simulink model "ddc_bpm_476_066"  (Simulink 7.8)
settings: Solver=ode45  StartTime=0.0  StopTime=0.012  RelTol=1e-3
undefined symbols (not defined in the file): dt_sim, frev_476, Fs_adc, xlipgetpartsetting
libraries: xbsIndex_r4 x601, simulink x5
(part 4 of 6)

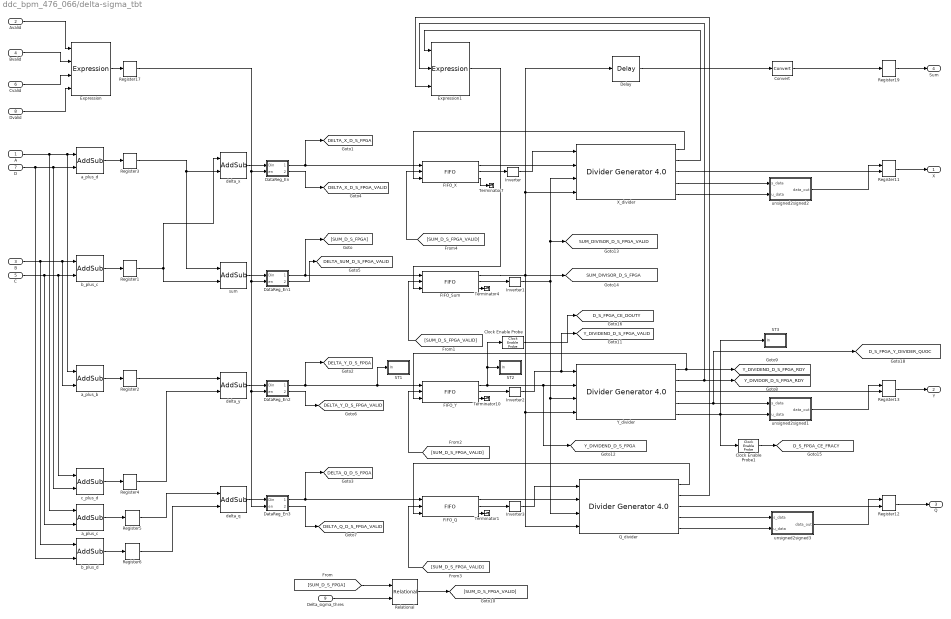
== system ddc_bpm_476_066/delta-sigma_tbt ==
  A : Inport
  Avalid : Inport  Port=2
  B : Inport  Port=3
  Bvalid : Inport  Port=4
  C : Inport  Port=5
  Cvalid : Inport  Port=6
  D : Inport  Port=7
  Dvalid : Inport  Port=8
  Delta_sigma_thres : Inport  Port=9
  Clock Enable Probe : xbsIndex_r4/Clock Enable Probe  inherit_constraints=on  block_type=ceprobe
      settings: infoedit="Clock enable extractor.  Produces a Boolean output that mirrors the hardware clock enable associated with the input sample rate.<br><br>Hardware notes: in hardware this block costs nothing."
  Clock Enable Probe1 : xbsIndex_r4/Clock Enable Probe  inherit_constraints=on  block_type=ceprobe
      settings: infoedit="Clock enable extractor.  Produces a Boolean output that mirrors the hardware clock enable associated with the input sample rate.<br><br>Hardware notes: in hardware this block costs nothing."
  Convert : xbsIndex_r4/Convert  gui_display_data_type=Fixed-point  arith_type="Signed  (2's comp)"  n_bits=24  bin_pt=20  float_type=Single  exp_bits=8  fraction_bits=24  quantization="Round  (unbiased: +/- Inf)"  overflow=Flag as error  en=off  latency=0  dbl_ovrd=off  pipeline=off  block_type=convert
  DataReg_En : Subsystem
  DataReg_En1 : Subsystem
  DataReg_En2 : Subsystem
  DataReg_En3 : Subsystem
  Delay : xbsIndex_r4/Delay  rst=off  infoeditControl=Selection of Reset will increase slice count due to use of real FFs and instead of SRLs  en=off  latency=39  dbl_ovrd=off  reg_retiming=off  block_type=delay
  Expression : xbsIndex_r4/Expression  expression=a & b & c & d  align_bp=on  en=off  latency=0  precision=Full  arith_type=Unsigned  n_bits=16  bin_pt=0  dbl_ovrd=off  block_type=expr
  Expression1 : xbsIndex_r4/Expression  expression=a & b & c  align_bp=on  en=off  latency=0  precision=Full  arith_type=Unsigned  n_bits=16  bin_pt=0  dbl_ovrd=off  block_type=expr
  FIFO_Q : xbsIndex_r4/FIFO  performance_options=First_Word_Fall_Through  depth=32  percent_nbits=1  rst=off  en=off  use_dcount=off  use_percent_full_port=off  use_almost_empty=off  almost_empty_thresh=2  use_almost_full=off  almost_full_thresh=14  dbl_ovrd=off  mem_type=Distributed RAM  explicit_period=off  block_type=fifo
  FIFO_Sum : xbsIndex_r4/FIFO  performance_options=First_Word_Fall_Through  depth=32  percent_nbits=1  rst=off  en=off  use_dcount=off  use_percent_full_port=off  use_almost_empty=off  almost_empty_thresh=2  use_almost_full=off  almost_full_thresh=14  dbl_ovrd=off  mem_type=Distributed RAM  explicit_period=off  block_type=fifo
  FIFO_X : xbsIndex_r4/FIFO  performance_options=First_Word_Fall_Through  depth=32  percent_nbits=1  rst=off  en=off  use_dcount=off  use_percent_full_port=off  use_almost_empty=off  almost_empty_thresh=2  use_almost_full=off  almost_full_thresh=14  dbl_ovrd=off  mem_type=Distributed RAM  explicit_period=off  block_type=fifo
  FIFO_Y : xbsIndex_r4/FIFO  performance_options=First_Word_Fall_Through  depth=32  percent_nbits=1  rst=off  en=off  use_dcount=off  use_percent_full_port=off  use_almost_empty=off  almost_empty_thresh=2  use_almost_full=off  almost_full_thresh=14  dbl_ovrd=off  mem_type=Distributed RAM  explicit_period=off  block_type=fifo
  Inverter{,1..3} (4 alike) : xbsIndex_r4/Inverter  en=off  latency=0  dbl_ovrd=off  block_type=inv
  Q_divider : xbsIndex_r4/Divider Generator 4.0   algorithm_type=High_Radix  remainder_type=Fractional  fractional_width=23  clocks_per_division=1  divide_by_zero_detect=off  flowcontrol=NonBlocking  optimizegoal=Performance  latency_configuration=Automatic  latency=39  dividend_has_tuser=off  dividend_has_tlast=off  divisor_has_tuser=off  divisor_has_tlast=off  aclken=off  aresetn=off  outtready=off  outtlastbehv=Null  trim_axipin_name=on  dividend_tuser_width=1  divisor_tuser_width=1  operand_sign=Signed  dividend_and_quotient_width=16  divisor_width=16  ip_name=Divider Generator  ip_version=4.0  dsptool_ready=true  ipcore_usecache=true  ipcore_useipmodelcache=true  wrapper_available=true  port_translation_map={'aclken' => 'en','aresetn' => 'rst'}  ipcore_fpga_part=xlipgetpartsetting(gcb, {'virtex7', 'xc7v1500t', '-2', 'fhg1157'})  ipcore_verbose=false  block_type=div_gen_v4_0
      settings: infoedit=Divider Generator 4.0
  Register{1..6,17,19} (8 alike) : xbsIndex_r4/Register  init=0  rst=off  en=off  dbl_ovrd=off  block_type=register
  Register11 : xbsIndex_r4/Register  init=0  rst=off  en=on  dbl_ovrd=off  block_type=register
  Register12 : xbsIndex_r4/Register  init=0  rst=off  en=on  dbl_ovrd=off  block_type=register
  Register13 : xbsIndex_r4/Register  init=0  rst=off  en=on  dbl_ovrd=off  block_type=register
  Relational : xbsIndex_r4/Relational  mode=a>b  en=off  latency=0  dbl_ovrd=off  block_type=relational
  ST1 : Subsystem
  ST2 : Subsystem
  ST3 : Subsystem
  Terminator{1,4,7,10} (4 alike) : Terminator
  X_divider : xbsIndex_r4/Divider Generator 4.0   algorithm_type=High_Radix  remainder_type=Fractional  fractional_width=23  clocks_per_division=1  divide_by_zero_detect=off  flowcontrol=NonBlocking  optimizegoal=Performance  latency_configuration=Automatic  latency=39  dividend_has_tuser=off  dividend_has_tlast=off  divisor_has_tuser=off  divisor_has_tlast=off  aclken=off  aresetn=off  outtready=off  outtlastbehv=Null  trim_axipin_name=on  dividend_tuser_width=1  divisor_tuser_width=1  operand_sign=Signed  dividend_and_quotient_width=16  divisor_width=16  ip_name=Divider Generator  ip_version=4.0  dsptool_ready=true  ipcore_usecache=true  ipcore_useipmodelcache=true  wrapper_available=true  port_translation_map={'aclken' => 'en','aresetn' => 'rst'}  ipcore_fpga_part=xlipgetpartsetting(gcb, {'virtex7', 'xc7v1500t', '-2', 'fhg1157'})  ipcore_verbose=false  block_type=div_gen_v4_0
      settings: infoedit=Divider Generator 4.0
  Y_divider : xbsIndex_r4/Divider Generator 4.0   algorithm_type=High_Radix  remainder_type=Fractional  fractional_width=23  clocks_per_division=1  divide_by_zero_detect=off  flowcontrol=NonBlocking  optimizegoal=Performance  latency_configuration=Automatic  latency=39  dividend_has_tuser=off  dividend_has_tlast=off  divisor_has_tuser=off  divisor_has_tlast=off  aclken=off  aresetn=off  outtready=off  outtlastbehv=Null  trim_axipin_name=on  dividend_tuser_width=1  divisor_tuser_width=1  operand_sign=Signed  dividend_and_quotient_width=16  divisor_width=16  ip_name=Divider Generator  ip_version=4.0  dsptool_ready=true  ipcore_usecache=true  ipcore_useipmodelcache=true  wrapper_available=true  port_translation_map={'aclken' => 'en','aresetn' => 'rst'}  ipcore_fpga_part=xlipgetpartsetting(gcb, {'virtex7', 'xc7v1500t', '-2', 'fhg1157'})  ipcore_verbose=false  block_type=div_gen_v4_0
      settings: infoedit=Divider Generator 4.0
  a_plus_b : xbsIndex_r4/AddSub  mode=Addition  use_carryin=off  use_carryout=off  en=off  latency=0  precision=Full  arith_type=Unsigned  n_bits=16  bin_pt=14  quantization=Truncate  overflow=Wrap  dbl_ovrd=off  use_behavioral_HDL=off  hw_selection=Fabric  pipelined=off  block_type=addsub
  a_plus_c : xbsIndex_r4/AddSub  mode=Addition  use_carryin=off  use_carryout=off  en=off  latency=0  precision=Full  arith_type=Unsigned  n_bits=16  bin_pt=14  quantization=Truncate  overflow=Wrap  dbl_ovrd=off  use_behavioral_HDL=off  hw_selection=Fabric  pipelined=off  block_type=addsub
  a_plus_d : xbsIndex_r4/AddSub  mode=Addition  use_carryin=off  use_carryout=off  en=off  latency=0  precision=Full  arith_type=Unsigned  n_bits=16  bin_pt=14  quantization=Truncate  overflow=Wrap  dbl_ovrd=off  use_behavioral_HDL=off  hw_selection=Fabric  pipelined=off  block_type=addsub
  b_plus_c : xbsIndex_r4/AddSub  mode=Addition  use_carryin=off  use_carryout=off  en=off  latency=0  precision=Full  arith_type=Unsigned  n_bits=16  bin_pt=14  quantization=Truncate  overflow=Wrap  dbl_ovrd=off  use_behavioral_HDL=off  hw_selection=Fabric  pipelined=off  block_type=addsub
  b_plus_d : xbsIndex_r4/AddSub  mode=Addition  use_carryin=off  use_carryout=off  en=off  latency=0  precision=Full  arith_type=Unsigned  n_bits=16  bin_pt=14  quantization=Truncate  overflow=Wrap  dbl_ovrd=off  use_behavioral_HDL=off  hw_selection=Fabric  pipelined=off  block_type=addsub
  c_plus_d : xbsIndex_r4/AddSub  mode=Addition  use_carryin=off  use_carryout=off  en=off  latency=0  precision=Full  arith_type=Unsigned  n_bits=16  bin_pt=14  quantization=Truncate  overflow=Wrap  dbl_ovrd=off  use_behavioral_HDL=off  hw_selection=Fabric  pipelined=off  block_type=addsub
  delta_q : xbsIndex_r4/AddSub  mode=Subtraction  use_carryin=off  use_carryout=off  en=off  latency=0  precision=Full  arith_type=Unsigned  n_bits=16  bin_pt=14  quantization=Truncate  overflow=Wrap  dbl_ovrd=off  use_behavioral_HDL=off  hw_selection=Fabric  pipelined=off  block_type=addsub
  delta_x : xbsIndex_r4/AddSub  mode=Subtraction  use_carryin=off  use_carryout=off  en=off  latency=0  precision=Full  arith_type=Unsigned  n_bits=16  bin_pt=14  quantization=Truncate  overflow=Wrap  dbl_ovrd=off  use_behavioral_HDL=off  hw_selection=Fabric  pipelined=off  block_type=addsub
  delta_y : xbsIndex_r4/AddSub  mode=Subtraction  use_carryin=off  use_carryout=off  en=off  latency=0  precision=Full  arith_type=Unsigned  n_bits=16  bin_pt=14  quantization=Truncate  overflow=Wrap  dbl_ovrd=off  use_behavioral_HDL=off  hw_selection=Fabric  pipelined=off  block_type=addsub
  sum : xbsIndex_r4/AddSub  mode=Addition  use_carryin=off  use_carryout=off  en=off  latency=0  precision=Full  arith_type=Unsigned  n_bits=16  bin_pt=14  quantization=Truncate  overflow=Wrap  dbl_ovrd=off  use_behavioral_HDL=off  hw_selection=Fabric  pipelined=off  block_type=addsub
  unsigned2signed1 : Subsystem
  unsigned2signed2 : Subsystem
  unsigned2signed3 : Subsystem
  X : Outport
  Y : Outport  Port=2
  Q : Outport  Port=3
  Sum : Outport  Port=4
  tag scope: DELTA_Q_D_S_FPGA=global, DELTA_Q_D_S_FPGA_VALID=global, DELTA_SUM_D_S_FPGA_VALID=global, DELTA_X_D_S_FPGA=global, DELTA_X_D_S_FPGA_VALID=global, DELTA_Y_D_S_FPGA=global, DELTA_Y_D_S_FPGA_VALID=global, D_S_FPGA_CE_DOUTY=global, D_S_FPGA_CE_FRACY=global, D_S_FPGA_Y_DIVIDER_QUOC=global, SUM_DIVISOR_D_S_FPGA=global, SUM_DIVISOR_D_S_FPGA_VALID=global, Y_DIVIDEND_D_S_FPGA=global, Y_DIVIDEND_D_S_FPGA_RDY=global, Y_DIVIDEND_D_S_FPGA_VALID=global, Y_DIVIDOR_D_S_FPGA_RDY=global
  wires:
  A/1 -> a_plus_d/1, a_plus_b/1, a_plus_c/1
  D/1 -> a_plus_d/2, c_plus_d/2, b_plus_d/2
  B/1 -> b_plus_c/1, a_plus_b/2, b_plus_d/1
  C/1 -> b_plus_c/2, c_plus_d/1, a_plus_c/2
  a_plus_d/1 -> Register3/1
  b_plus_c/1 -> Register1/1
  a_plus_b/1 -> Register2/1
  c_plus_d/1 -> Register4/1
  a_plus_c/1 -> Register5/1
  b_plus_d/1 -> Register6/1
  Register3/1 -> sum/1, delta_x/2
  Register1/1 -> sum/2, delta_x/1
  Register2/1 -> delta_y/1
  Register4/1 -> delta_y/2
  Register5/1 -> delta_q/1
  Register6/1 -> delta_q/2
  delta_q/1 -> DataReg_En3/1(Din)
  delta_x/1 -> DataReg_En/1(Din)
  Register19/1 -> Sum/1
  Avalid/1 -> Expression/1
  Bvalid/1 -> Expression/2
  Cvalid/1 -> Expression/3
  Dvalid/1 -> Expression/4
  Expression/1 -> Register17/1
  DataReg_En1/1(Dout) -> [SUM_D_S_FPGA], FIFO_Sum/1
  Register17/1 -> DataReg_En/2(en), DataReg_En1/2(en), DataReg_En2/2(en), DataReg_En3/2(en)
  Register13/1 -> Y/1
  Register11/1 -> X/1
  Register12/1 -> Q/1
  sum/1 -> DataReg_En1/1(Din)
  delta_y/1 -> DataReg_En2/1(Din)
  DataReg_En1/2(Valid) -> [DELTA_SUM_D_S_FPGA_VALID]
  Delay/1 -> Convert/1
  X_divider/3 -> Register11/2
  DataReg_En/1(Dout) -> [DELTA_X_D_S_FPGA], FIFO_X/1
  DataReg_En/2(Valid) -> [DELTA_X_D_S_FPGA_VALID]
  Y_divider/5 -> ST3/1(In), Clock Enable Probe1/1, unsigned2signed1/2(u_data)
  Y_divider/3 -> Register13/2
  Q_divider/3 -> Register12/2
  DataReg_En2/1(Dout) -> [DELTA_Y_D_S_FPGA], FIFO_Y/1, ST1/1(In)
  DataReg_En2/2(Valid) -> [DELTA_Y_D_S_FPGA_VALID]
  DataReg_En3/1(Dout) -> [DELTA_Q_D_S_FPGA], FIFO_Q/1
  DataReg_En3/2(Valid) -> [DELTA_Q_D_S_FPGA_VALID]
  X_divider/2 -> Expression1/1
  Y_divider/1 -> [Y_DIVIDEND_D_S_FPGA_RDY], FIFO_Y/3
  Y_divider/2 -> [Y_DIVIDOR_D_S_FPGA_RDY], Expression1/2
  Delta_sigma_thres/1 -> Relational/2
  [SUM_D_S_FPGA] -> Relational/1
  Relational/1 -> [SUM_D_S_FPGA_VALID]
  [SUM_D_S_FPGA_VALID] -> FIFO_Sum/2
  FIFO_Sum/1 -> Y_divider/4, Q_divider/4, X_divider/4, Delay/1, [SUM_DIVISOR_D_S_FPGA]
  FIFO_X/1 -> X_divider/2
  FIFO_Q/1 -> Q_divider/2
  FIFO_Y/1 -> Y_divider/2, [Y_DIVIDEND_D_S_FPGA], ST2/1(In), Clock Enable Probe/1
  Q_divider/2 -> Expression1/3
  Expression1/1 -> FIFO_Sum/3
  X_divider/1 -> FIFO_X/3
  Q_divider/1 -> FIFO_Q/3
  [SUM_D_S_FPGA_VALID] -> FIFO_Y/2
  [SUM_D_S_FPGA_VALID] -> FIFO_Q/2
  FIFO_Q/2 -> Inverter3/1
  FIFO_Q/3 -> Terminator1/1
  FIFO_Sum/2 -> Inverter1/1
  FIFO_Sum/3 -> Terminator4/1
  FIFO_X/3 -> Terminator7/1
  FIFO_Y/2 -> Inverter2/1
  FIFO_Y/3 -> Terminator10/1
  [SUM_D_S_FPGA_VALID] -> FIFO_X/2
  FIFO_X/2 -> Inverter/1
  Inverter/1 -> X_divider/1
  Inverter1/1 -> Y_divider/3, Q_divider/3, X_divider/3, [SUM_DIVISOR_D_S_FPGA_VALID]
  Inverter2/1 -> Y_divider/1, [Y_DIVIDEND_D_S_FPGA_VALID]
  Inverter3/1 -> Q_divider/1
  Clock Enable Probe1/1 -> [D_S_FPGA_CE_FRACY]
  Clock Enable Probe/1 -> [D_S_FPGA_CE_DOUTY]
  X_divider/5 -> unsigned2signed2/2(u_data)
  X_divider/4 -> unsigned2signed2/1(s_data)
  unsigned2signed2/1(data_out) -> Register11/1
  Y_divider/4 -> [D_S_FPGA_Y_DIVIDER_QUOC], unsigned2signed1/1(s_data)
  unsigned2signed1/1(data_out) -> Register13/1
  Q_divider/5 -> unsigned2signed3/2(u_data)
  Q_divider/4 -> unsigned2signed3/1(s_data)
  unsigned2signed3/1(data_out) -> Register12/1
  Convert/1 -> Register19/1

== system ddc_bpm_476_066/BPF/Cast ==
  data_in : Inport
  en : Inport  Port=2
  Convert : xbsIndex_r4/Convert  gui_display_data_type=Fixed-point  arith_type="Signed  (2's comp)"  n_bits=24  bin_pt=22  float_type=Single  exp_bits=8  fraction_bits=24  quantization="Round  (unbiased: +/- Inf)"  overflow=Flag as error  en=off  latency=0  dbl_ovrd=off  pipeline=off  block_type=convert
      settings: xl_area=[0, 0, 0, 0, 0, 0, 0]  block_version=VER_STRING_GOES_HERE
  Register : xbsIndex_r4/Register  init=0  rst=off  en=on  dbl_ovrd=off  block_type=register
      settings: xl_area=[0, 0, 0, 0, 0, 0, 0]  block_version=VER_STRING_GOES_HERE
  out : Outport  SampleTime=dt_sim
  wires:
  Convert/1 -> Register/1
  Register/1 -> out/1
  en/1 -> Register/2
  data_in/1 -> Convert/1

== system ddc_bpm_476_066/BPF/Cast1 ==
  data_in : Inport
  en : Inport  Port=2
  Convert : xbsIndex_r4/Convert  gui_display_data_type=Fixed-point  arith_type="Signed  (2's comp)"  n_bits=24  bin_pt=22  float_type=Single  exp_bits=8  fraction_bits=24  quantization="Round  (unbiased: +/- Inf)"  overflow=Flag as error  en=off  latency=0  dbl_ovrd=off  pipeline=off  block_type=convert
      settings: xl_area=[0, 0, 0, 0, 0, 0, 0]  block_version=VER_STRING_GOES_HERE
  Register : xbsIndex_r4/Register  init=0  rst=off  en=on  dbl_ovrd=off  block_type=register
      settings: xl_area=[0, 0, 0, 0, 0, 0, 0]  block_version=VER_STRING_GOES_HERE
  out : Outport  SampleTime=dt_sim
  wires:
  Convert/1 -> Register/1
  Register/1 -> out/1
  en/1 -> Register/2
  data_in/1 -> Convert/1

== system ddc_bpm_476_066/BPF/Cast2 ==
  data_in : Inport
  en : Inport  Port=2
  Convert : xbsIndex_r4/Convert  gui_display_data_type=Fixed-point  arith_type="Signed  (2's comp)"  n_bits=24  bin_pt=22  float_type=Single  exp_bits=8  fraction_bits=24  quantization="Round  (unbiased: +/- Inf)"  overflow=Flag as error  en=off  latency=0  dbl_ovrd=off  pipeline=off  block_type=convert
      settings: xl_area=[0, 0, 0, 0, 0, 0, 0]  block_version=VER_STRING_GOES_HERE
  Register : xbsIndex_r4/Register  init=0  rst=off  en=on  dbl_ovrd=off  block_type=register
      settings: xl_area=[0, 0, 0, 0, 0, 0, 0]  block_version=VER_STRING_GOES_HERE
  out : Outport  SampleTime=dt_sim
  wires:
  Convert/1 -> Register/1
  Register/1 -> out/1
  en/1 -> Register/2
  data_in/1 -> Convert/1

== system ddc_bpm_476_066/BPF/Cast3 ==
  data_in : Inport
  en : Inport  Port=2
  Convert : xbsIndex_r4/Convert  gui_display_data_type=Fixed-point  arith_type="Signed  (2's comp)"  n_bits=24  bin_pt=22  float_type=Single  exp_bits=8  fraction_bits=24  quantization="Round  (unbiased: +/- Inf)"  overflow=Flag as error  en=off  latency=0  dbl_ovrd=off  pipeline=off  block_type=convert
      settings: xl_area=[0, 0, 0, 0, 0, 0, 0]  block_version=VER_STRING_GOES_HERE
  Register : xbsIndex_r4/Register  init=0  rst=off  en=on  dbl_ovrd=off  block_type=register
      settings: xl_area=[0, 0, 0, 0, 0, 0, 0]  block_version=VER_STRING_GOES_HERE
  out : Outport  SampleTime=dt_sim
  wires:
  Convert/1 -> Register/1
  Register/1 -> out/1
  en/1 -> Register/2
  data_in/1 -> Convert/1

== system ddc_bpm_476_066/Channel0_fofb/Analysis ==
  CIC_FOFB : Scope  NumInputPorts=2
      settings: TimeRange=0.00011214  YMin=-0.243948~-0.279234  YMax=-0.220714~-0.25264  SaveName=ScopeData4  MaxDataPoints=1000000  SampleInput=on
  CORDIC_FOFB : Scope  NumInputPorts=2
      settings: TimeRange=0.00011214  YMin=0.475054~-10  YMax=0.52506~45  SaveName=ScopeData5  MaxDataPoints=1000000  SampleInput=on
  bpf_ch0_o{5..8} (4 alike) : xbsIndex_r4/Gateway Out  inherit_from_input=on  hdl_port=off  timing_constraint=Data Rate  locs_specified=off  LOCs={}  UseAsDAC=off  DACChannel='1'  block_type=gatewayout
      settings: infoedit="Gateway out block.  Converts Xilinx fixed-point or floating-point type inputs into ouputs of type Simulink integer, single, double, or fixed point.<br><br>Hardware notes:  In hardware these blocks become top level output ports or are discarded, depending on how they are configured."
  wires:
  bpf_ch0_o5/1 -> CIC_FOFB/1
  [CIC_FOFB_I_FPGA_OUT] -> bpf_ch0_o5/1
  bpf_ch0_o6/1 -> CIC_FOFB/2
  [CIC_FOFB_Q_FPGA_OUT] -> bpf_ch0_o6/1
  bpf_ch0_o7/1 -> CORDIC_FOFB/1
  [CORDIC_FOFB_R_FPGA_OUT] -> bpf_ch0_o7/1
  bpf_ch0_o8/1 -> CORDIC_FOFB/2
  [CORDIC_FOFB_T_FPGA_OUT] -> bpf_ch0_o8/1

== system ddc_bpm_476_066/Channel0_fofb/cic_fofb ==
  Q_in : Inport
  I_in : Inport  Port=2
  Reinterpret : xbsIndex_r4/Reinterpret  force_arith_type=on  arith_type="Signed  (2's comp)"  force_bin_pt=on  bin_pt=22  block_type=reinterpret
  Reinterpret1 : xbsIndex_r4/Reinterpret  force_arith_type=on  arith_type="Signed  (2's comp)"  force_bin_pt=on  bin_pt=22  block_type=reinterpret
  Terminator : Terminator
  Terminator1 : Terminator
  cic_fofb_i : xbsIndex_r4/CIC Compiler 3.0   filter_type=Decimation  number_of_stages=5  differential_delay=2  number_of_channels=1  sample_rate_changes=Fixed  fixed_or_initial_rate=R_fofb  minimum_rate=1113  maximum_rate=1113  ratespecification=Maximum_Possible  sampleperiod=1  hardwareoversamplingrate=1  quantization=Truncation  output_data_width=24  use_xtreme_dsp_slice=on  use_streaming_interface=on  has_aclken=off  has_aresetn=off  has_dout_tready=off  trim_axipin_name=on  gui_behaviour=Sysgen_GUI  input_data_width=18  ip_name=CIC Compiler  ip_version=3.0  dsptool_ready=true  wrapper_available=true  port_translation_map={ 'aclken' => 'en', 'aresetn' => 'rst' }  ipcore_xco_need_fpga_part=true  ipcore_fpga_part=xlipgetpartsetting(gcb, {'virtex7', 'xc7v1500t', '-2', 'fhg1157'})  ipcore_verbose=false  block_type=cic_compiler_v3_0
  cic_fofb_q : xbsIndex_r4/CIC Compiler 3.0   filter_type=Decimation  number_of_stages=5  differential_delay=2  number_of_channels=1  sample_rate_changes=Fixed  fixed_or_initial_rate=R_fofb  minimum_rate=1113  maximum_rate=1113  ratespecification=Maximum_Possible  sampleperiod=1  hardwareoversamplingrate=1  quantization=Truncation  output_data_width=24  use_xtreme_dsp_slice=on  use_streaming_interface=on  has_aclken=off  has_aresetn=off  has_dout_tready=off  trim_axipin_name=on  gui_behaviour=Sysgen_GUI  input_data_width=18  ip_name=CIC Compiler  ip_version=3.0  dsptool_ready=true  wrapper_available=true  port_translation_map={ 'aclken' => 'en', 'aresetn' => 'rst' }  ipcore_xco_need_fpga_part=true  ipcore_fpga_part=xlipgetpartsetting(gcb, {'virtex7', 'xc7v1500t', '-2', 'fhg1157'})  ipcore_verbose=false  block_type=cic_compiler_v3_0
  Q_out : Outport
  Q_valid : Outport  Port=2
  I_out : Outport  Port=3
  I_valid : Outport  Port=4
  wires:
  I_in/1 -> cic_fofb_i/1
  cic_fofb_i/2 -> I_valid/1
  Q_in/1 -> cic_fofb_q/1
  cic_fofb_q/2 -> Q_valid/1
  cic_fofb_i/1 -> Terminator/1
  cic_fofb_q/1 -> Terminator1/1
  Reinterpret/1 -> Q_out/1
  cic_fofb_q/3 -> Reinterpret/1
  Reinterpret1/1 -> I_out/1
  cic_fofb_i/3 -> Reinterpret1/1

== system ddc_bpm_476_066/Channel0_tbt/Analysis ==
  ADC_in1 : Scope
      settings: TimeRange=0.00011214  YMin=-0.1  YMax=0.1  MaxDataPoints=1000000  SampleInput=on
  CORDIC : Scope  NumInputPorts=2
      settings: TimeRange=0.00011214  YMin=0.475054~-10  YMax=0.52506~45  SaveName=ScopeData5  MaxDataPoints=1000000  SampleInput=on
  DECIM_35 : Scope  NumInputPorts=2
      settings: TimeRange=0.00011214  YMin=0.440352~-0.0607492  YMax=0.440353~-0.060745  SaveName=ScopeData4  MaxDataPoints=1000000  SampleInput=on
  MIX : Scope  NumInputPorts=4
      settings: TimeRange=0.00011214  YMin=-0.1~-1.5~-0.002~-1.5  YMax=1~1.5~0.00075~1.5  SaveName=ScopeData2  MaxDataPoints=1000000  SampleInput=on
  bpf_ch0_o{1,3..10} (9 alike) : xbsIndex_r4/Gateway Out  inherit_from_input=on  hdl_port=off  timing_constraint=Data Rate  locs_specified=off  LOCs={}  UseAsDAC=off  DACChannel='1'  block_type=gatewayout
      settings: infoedit="Gateway out block.  Converts Xilinx fixed-point or floating-point type inputs into ouputs of type Simulink integer, single, double, or fixed point.<br><br>Hardware notes:  In hardware these blocks become top level output ports or are discarded, depending on how they are configured."
  wires:
  [BPF_IN] -> bpf_ch0_o1/1
  bpf_ch0_o3/1 -> MIX/1
  [MIX_I_FPGA_OUT] -> bpf_ch0_o3/1
  [MIX_Q_FPGA_OUT] -> bpf_ch0_o4/1
  bpf_ch0_o4/1 -> MIX/3
  [DDS_MSIN_FPGA_OUT] -> bpf_ch0_o9/1
  bpf_ch0_o9/1 -> MIX/2
  [DDS_COS_FPGA_OUT] -> bpf_ch0_o10/1
  bpf_ch0_o10/1 -> MIX/4
  bpf_ch0_o5/1 -> DECIM_35/1
  [DECIM_35_I_FPGA_OUT] -> bpf_ch0_o5/1
  bpf_ch0_o6/1 -> DECIM_35/2
  [DECIM_35_Q_FPGA_OUT] -> bpf_ch0_o6/1
  bpf_ch0_o7/1 -> CORDIC/1
  [CORDIC_R_FPGA_OUT] -> bpf_ch0_o7/1
  bpf_ch0_o8/1 -> CORDIC/2
  [CORDIC_T_FPGA_OUT] -> bpf_ch0_o8/1
  bpf_ch0_o1/1 -> ADC_in1/1

== system ddc_bpm_476_066/Channel0_tbt/DDC ==
  data_in : Inport
  DDS_msine_in : Inport  Port=2
  DDS_cosine_in : Inport  Port=3
  DDS_valid_in : Inport  Port=4
  Constant1 : xbsIndex_r4/Constant  const=1  gui_display_data_type=Boolean  arith_type=Boolean  n_bits=24  bin_pt=22  preci_type=Single  exp_width=8  frac_width=24  explicit_period=on  period=dt_sim  equ=P=C  opselect=C  inp2=PCIN>>17  opr=+  inp1=P  carry=CIN  dbl_ovrd=off  block_type=constant
  Constant2 : xbsIndex_r4/Constant  const=0  gui_display_data_type=Fixed-point  arith_type=Signed (2's comp)  n_bits=24  bin_pt=22  preci_type=Single  exp_width=8  frac_width=24  explicit_period=on  period=dt_sim  equ=P=C  opselect=C  inp2=PCIN>>17  opr=+  inp1=P  carry=CIN  dbl_ovrd=off  block_type=constant
  Mixer : Subsystem
  mix_q_out : Outport
  mix_i_out : Outport  Port=2
  valid_out : Outport  Port=3
  wires:
  Constant1/1 -> Mixer/3(en)
  Constant2/1 -> Mixer/1(din_q)
  DDS_valid_in/1 -> Mixer/4(dds_valid)
  DDS_cosine_in/1 -> Mixer/5(dds_cosine)
  DDS_msine_in/1 -> Mixer/6(dds_msine)
  data_in/1 -> Mixer/2(din_i)
  Mixer/1(Q) -> mix_q_out/1
  Mixer/2(I) -> mix_i_out/1
  Mixer/3(valid_out) -> valid_out/1

== system ddc_bpm_476_066/Channel0_tbt/decim35 ==
  Q_in : Inport
  I_in : Inport  Port=2
  Cast1 : Subsystem
  Cast4 : Subsystem
  "FIR Compiler 6.2 " : xbsIndex_r4/FIR Compiler 6.2   coefficientvector=Hpoly_35.Numerator  coefficient_sets=1  filter_type=Decimation  rate_change_type=Integer  interpolation_rate=1  decimation_rate=decim_factor_poly_35  number_channels=1  ratespecification=Maximum_Possible  sampleperiod=1  hardwareoversamplingrate=4  filter_architecture=Systolic_Multiply_Accumulate  coefficient_reload=off  coefficient_sign=Signed  quantization=Quantize_Only  coefficient_width=16  bestprecision=on  coefficient_fractional_bits=20  coefficient_structure=Inferred  number_paths=2  output_rounding_mode=Convergent_Rounding_to_Even  output_width=24  optimization_goal=Area  data_has_tlast=Not_Required  m_data_has_tready=off  s_data_has_fifo=off  s_data_has_tuser=Not_Required  m_data_has_tuser=Not_Required  s_config_sync_mode=On_Vector  s_config_method=Single  num_reload_slots=1  has_aclken=off  has_aresetn=off  multi_column_support=Disabled  columnconfig='14'  inter_column_pipe_length=4  data_buffer_type=Automatic  coefficient_buffer_type=Automatic  input_buffer_type=Automatic  output_buffer_type=Automatic  preference_for_other_storage=Automatic  trim_axipin_name=on  passband_min=0.0  passband_max=0.5  stopband_min=0.5  stopband_max=1.0  filter_selection=1  gui_behaviour=Sysgen_GUI  data_sign=Signed  data_width=16  data_fractional_bits=0  wrapper_available=true  ip_wrap_arbitrary_binary_point=true  ip_name=FIR Compiler  ip_version=6.2  dsptool_ready=true  ipcore_usecache=true  ipcore_useipmodelcache=true  ipcore_xco_need_fpga_part=true  port_translation_map={ 'aclken' => 'en', 'aresetn' => 'rst' }  run_core_at_system_period=true  ipcore_fpga_part=xlipgetpartsetting(gcb, {'virtex6', 'xc6vlx75t', '-3', 'ff784'})  structural_sim=false  block_type=fir_compiler_v6_2
      settings: infoedit=Maximum Possible : Maximizes oversampling rate. Abstracted input handshake (no s_data_tvalid) and automatic rate propagation.<br>Hardware Oversampling Rate : Specifies oversampling rate relative to the input sample period. Abstracted input handshake (no s_data_tvalid) and automatic rate propagation.<br>Sample Period : Specifies absolute oversampling rate. No input handshake abstraction (exposes s_data_tvalid) and no rate propagation.
  Terminator : Terminator
  Terminator1 : Terminator
  Q_out : Outport
  I_out : Outport  Port=2
  valid_out : Outport  Port=3
  wires:
  Q_in/1 -> "FIR Compiler 6.2 "/1
  "FIR Compiler 6.2 "/2 -> Cast4/2(en), Cast1/2(en)
  "FIR Compiler 6.2 "/3 -> Cast4/1(data_in)
  Cast4/1(out) -> Q_out/1
  "FIR Compiler 6.2 "/4 -> Cast1/1(data_in)
  Cast1/1(out) -> I_out/1
  I_in/1 -> "FIR Compiler 6.2 "/2
  "FIR Compiler 6.2 "/1 -> Terminator/1
  Cast4/2(valid) -> valid_out/1
  Cast1/2(valid) -> Terminator1/1

== system ddc_bpm_476_066/Channel1_fofb/Analysis ==
  CIC_FOFB : Scope  NumInputPorts=2
      settings: TimeRange=0.00011214  YMin=0.440352~-0.0607492  YMax=0.440353~-0.060745  SaveName=ScopeData4  MaxDataPoints=1000000  SampleInput=on
  CORDIC_FOFB : Scope  NumInputPorts=2
      settings: TimeRange=0.00011214  YMin=0.475054~-10  YMax=0.52506~45  SaveName=ScopeData5  MaxDataPoints=1000000  SampleInput=on
  bpf_ch0_o{5..8} (4 alike) : xbsIndex_r4/Gateway Out  inherit_from_input=on  hdl_port=off  timing_constraint=Data Rate  locs_specified=off  LOCs={}  UseAsDAC=off  DACChannel='1'  block_type=gatewayout
      settings: infoedit="Gateway out block.  Converts Xilinx fixed-point or floating-point type inputs into ouputs of type Simulink integer, single, double, or fixed point.<br><br>Hardware notes:  In hardware these blocks become top level output ports or are discarded, depending on how they are configured."
  wires:
  bpf_ch0_o5/1 -> CIC_FOFB/1
  [CIC_FOFB_I_FPGA_OUT] -> bpf_ch0_o5/1
  bpf_ch0_o6/1 -> CIC_FOFB/2
  [CIC_FOFB_Q_FPGA_OUT] -> bpf_ch0_o6/1
  bpf_ch0_o7/1 -> CORDIC_FOFB/1
  [CORDIC_FOFB_R_FPGA_OUT] -> bpf_ch0_o7/1
  bpf_ch0_o8/1 -> CORDIC_FOFB/2
  [CORDIC_FOFB_T_FPGA_OUT] -> bpf_ch0_o8/1

== system ddc_bpm_476_066/Channel1_fofb/cic_fofb ==
  Q_in : Inport
  I_in : Inport  Port=2
  Reinterpret : xbsIndex_r4/Reinterpret  force_arith_type=on  arith_type="Signed  (2's comp)"  force_bin_pt=on  bin_pt=22  block_type=reinterpret
  Reinterpret1 : xbsIndex_r4/Reinterpret  force_arith_type=on  arith_type="Signed  (2's comp)"  force_bin_pt=on  bin_pt=22  block_type=reinterpret
  Terminator : Terminator
  Terminator1 : Terminator
  cic_fofb_i : xbsIndex_r4/CIC Compiler 3.0   filter_type=Decimation  number_of_stages=5  differential_delay=2  number_of_channels=1  sample_rate_changes=Fixed  fixed_or_initial_rate=R_fofb  minimum_rate=1113  maximum_rate=1113  ratespecification=Maximum_Possible  sampleperiod=1  hardwareoversamplingrate=1  quantization=Truncation  output_data_width=24  use_xtreme_dsp_slice=on  use_streaming_interface=on  has_aclken=off  has_aresetn=off  has_dout_tready=off  trim_axipin_name=on  gui_behaviour=Sysgen_GUI  input_data_width=18  ip_name=CIC Compiler  ip_version=3.0  dsptool_ready=true  wrapper_available=true  port_translation_map={ 'aclken' => 'en', 'aresetn' => 'rst' }  ipcore_xco_need_fpga_part=true  ipcore_fpga_part=xlipgetpartsetting(gcb, {'virtex7', 'xc7v1500t', '-2', 'fhg1157'})  ipcore_verbose=false  block_type=cic_compiler_v3_0
  cic_fofb_q : xbsIndex_r4/CIC Compiler 3.0   filter_type=Decimation  number_of_stages=5  differential_delay=2  number_of_channels=1  sample_rate_changes=Fixed  fixed_or_initial_rate=R_fofb  minimum_rate=1113  maximum_rate=1113  ratespecification=Maximum_Possible  sampleperiod=1  hardwareoversamplingrate=1  quantization=Truncation  output_data_width=24  use_xtreme_dsp_slice=on  use_streaming_interface=on  has_aclken=off  has_aresetn=off  has_dout_tready=off  trim_axipin_name=on  gui_behaviour=Sysgen_GUI  input_data_width=18  ip_name=CIC Compiler  ip_version=3.0  dsptool_ready=true  wrapper_available=true  port_translation_map={ 'aclken' => 'en', 'aresetn' => 'rst' }  ipcore_xco_need_fpga_part=true  ipcore_fpga_part=xlipgetpartsetting(gcb, {'virtex7', 'xc7v1500t', '-2', 'fhg1157'})  ipcore_verbose=false  block_type=cic_compiler_v3_0
  Q_out : Outport
  Q_valid : Outport  Port=2
  I_out : Outport  Port=3
  I_valid : Outport  Port=4
  wires:
  I_in/1 -> cic_fofb_i/1
  cic_fofb_i/2 -> I_valid/1
  Q_in/1 -> cic_fofb_q/1
  cic_fofb_q/2 -> Q_valid/1
  cic_fofb_i/1 -> Terminator/1
  cic_fofb_q/1 -> Terminator1/1
  Reinterpret/1 -> Q_out/1
  cic_fofb_q/3 -> Reinterpret/1
  Reinterpret1/1 -> I_out/1
  cic_fofb_i/3 -> Reinterpret1/1

== system ddc_bpm_476_066/Channel1_tbt/Analysis ==
  ADC_in1 : Scope
      settings: TimeRange=0.00011214  YMin=-0.1  YMax=0.1  MaxDataPoints=1000000  SampleInput=on
  CORDIC : Scope  NumInputPorts=2
      settings: TimeRange=0.00011214  YMin=0.475054~-10  YMax=0.52506~45  SaveName=ScopeData5  MaxDataPoints=1000000  SampleInput=on
  DECIM_35 : Scope  NumInputPorts=2
      settings: TimeRange=0.00011214  YMin=0.440352~-0.0607492  YMax=0.440353~-0.060745  SaveName=ScopeData4  MaxDataPoints=1000000  SampleInput=on
  MIX : Scope  NumInputPorts=4
      settings: TimeRange=0.00011214  YMin=-0.1~-1.5~-0.002~-1.5  YMax=1~1.5~0.00075~1.5  SaveName=ScopeData2  MaxDataPoints=1000000  SampleInput=on
  bpf_ch0_o{1,3..10} (9 alike) : xbsIndex_r4/Gateway Out  inherit_from_input=on  hdl_port=off  timing_constraint=Data Rate  locs_specified=off  LOCs={}  UseAsDAC=off  DACChannel='1'  block_type=gatewayout
      settings: infoedit="Gateway out block.  Converts Xilinx fixed-point or floating-point type inputs into ouputs of type Simulink integer, single, double, or fixed point.<br><br>Hardware notes:  In hardware these blocks become top level output ports or are discarded, depending on how they are configured."
  wires:
  [BPF_IN] -> bpf_ch0_o1/1
  bpf_ch0_o3/1 -> MIX/1
  [MIX_I_FPGA_OUT] -> bpf_ch0_o3/1
  [MIX_Q_FPGA_OUT] -> bpf_ch0_o4/1
  bpf_ch0_o4/1 -> MIX/3
  [DDS_MSIN_FPGA_OUT] -> bpf_ch0_o9/1
  bpf_ch0_o9/1 -> MIX/2
  [DDS_COS_FPGA_OUT] -> bpf_ch0_o10/1
  bpf_ch0_o10/1 -> MIX/4
  bpf_ch0_o5/1 -> DECIM_35/1
  [DECIM_35_I_FPGA_OUT] -> bpf_ch0_o5/1
  bpf_ch0_o6/1 -> DECIM_35/2
  [DECIM_35_Q_FPGA_OUT] -> bpf_ch0_o6/1
  bpf_ch0_o7/1 -> CORDIC/1
  [CORDIC_R_FPGA_OUT] -> bpf_ch0_o7/1
  bpf_ch0_o8/1 -> CORDIC/2
  [CORDIC_T_FPGA_OUT] -> bpf_ch0_o8/1
  bpf_ch0_o1/1 -> ADC_in1/1

== system ddc_bpm_476_066/Channel1_tbt/DDC ==
  data_in : Inport
  DDS_msine_in : Inport  Port=2
  DDS_cosine_in : Inport  Port=3
  DDS_valid_in : Inport  Port=4
  Constant1 : xbsIndex_r4/Constant  const=1  gui_display_data_type=Boolean  arith_type=Boolean  n_bits=24  bin_pt=22  preci_type=Single  exp_width=8  frac_width=24  explicit_period=on  period=dt_sim  equ=P=C  opselect=C  inp2=PCIN>>17  opr=+  inp1=P  carry=CIN  dbl_ovrd=off  block_type=constant
  Constant2 : xbsIndex_r4/Constant  const=0  gui_display_data_type=Fixed-point  arith_type=Signed (2's comp)  n_bits=24  bin_pt=22  preci_type=Single  exp_width=8  frac_width=24  explicit_period=on  period=dt_sim  equ=P=C  opselect=C  inp2=PCIN>>17  opr=+  inp1=P  carry=CIN  dbl_ovrd=off  block_type=constant
  Mixer : Subsystem
  mix_q_out : Outport
  mix_i_out : Outport  Port=2
  valid_out : Outport  Port=3
  wires:
  Constant1/1 -> Mixer/3(en)
  Constant2/1 -> Mixer/1(din_q)
  DDS_valid_in/1 -> Mixer/4(dds_valid)
  DDS_cosine_in/1 -> Mixer/5(dds_cosine)
  DDS_msine_in/1 -> Mixer/6(dds_msine)
  data_in/1 -> Mixer/2(din_i)
  Mixer/1(Q) -> mix_q_out/1
  Mixer/2(I) -> mix_i_out/1
  Mixer/3(valid_out) -> valid_out/1

== system ddc_bpm_476_066/Channel1_tbt/decim35 ==
  Q_in : Inport
  I_in : Inport  Port=2
  Cast1 : Subsystem
  Cast4 : Subsystem
  "FIR Compiler 6.2 " : xbsIndex_r4/FIR Compiler 6.2   coefficientvector=Hpoly_35.Numerator  coefficient_sets=1  filter_type=Decimation  rate_change_type=Integer  interpolation_rate=1  decimation_rate=decim_factor_poly_35  number_channels=1  ratespecification=Maximum_Possible  sampleperiod=1  hardwareoversamplingrate=4  filter_architecture=Systolic_Multiply_Accumulate  coefficient_reload=off  coefficient_sign=Signed  quantization=Quantize_Only  coefficient_width=16  bestprecision=on  coefficient_fractional_bits=20  coefficient_structure=Inferred  number_paths=2  output_rounding_mode=Convergent_Rounding_to_Even  output_width=24  optimization_goal=Area  data_has_tlast=Not_Required  m_data_has_tready=off  s_data_has_fifo=off  s_data_has_tuser=Not_Required  m_data_has_tuser=Not_Required  s_config_sync_mode=On_Vector  s_config_method=Single  num_reload_slots=1  has_aclken=off  has_aresetn=off  multi_column_support=Disabled  columnconfig='14'  inter_column_pipe_length=4  data_buffer_type=Automatic  coefficient_buffer_type=Automatic  input_buffer_type=Automatic  output_buffer_type=Automatic  preference_for_other_storage=Automatic  trim_axipin_name=on  passband_min=0.0  passband_max=0.5  stopband_min=0.5  stopband_max=1.0  filter_selection=1  gui_behaviour=Sysgen_GUI  data_sign=Signed  data_width=16  data_fractional_bits=0  wrapper_available=true  ip_wrap_arbitrary_binary_point=true  ip_name=FIR Compiler  ip_version=6.2  dsptool_ready=true  ipcore_usecache=true  ipcore_useipmodelcache=true  ipcore_xco_need_fpga_part=true  port_translation_map={ 'aclken' => 'en', 'aresetn' => 'rst' }  run_core_at_system_period=true  ipcore_fpga_part=xlipgetpartsetting(gcb, {'virtex6', 'xc6vlx75t', '-3', 'ff784'})  structural_sim=false  block_type=fir_compiler_v6_2
      settings: infoedit=Maximum Possible : Maximizes oversampling rate. Abstracted input handshake (no s_data_tvalid) and automatic rate propagation.<br>Hardware Oversampling Rate : Specifies oversampling rate relative to the input sample period. Abstracted input handshake (no s_data_tvalid) and automatic rate propagation.<br>Sample Period : Specifies absolute oversampling rate. No input handshake abstraction (exposes s_data_tvalid) and no rate propagation.
  Terminator : Terminator
  Terminator1 : Terminator
  Q_out : Outport
  I_out : Outport  Port=2
  valid_out : Outport  Port=3
  wires:
  Q_in/1 -> "FIR Compiler 6.2 "/1
  "FIR Compiler 6.2 "/2 -> Cast4/2(en), Cast1/2(en)
  "FIR Compiler 6.2 "/3 -> Cast4/1(data_in)
  Cast4/1(out) -> Q_out/1
  "FIR Compiler 6.2 "/4 -> Cast1/1(data_in)
  Cast1/1(out) -> I_out/1
  I_in/1 -> "FIR Compiler 6.2 "/2
  "FIR Compiler 6.2 "/1 -> Terminator/1
  Cast4/2(valid) -> valid_out/1
  Cast1/2(valid) -> Terminator1/1

== system ddc_bpm_476_066/Channel2_fofb/Analysis ==
  CIC_FOFB : Scope  NumInputPorts=2
      settings: TimeRange=0.00011214  YMin=0.440352~-0.0607492  YMax=0.440353~-0.060745  SaveName=ScopeData4  MaxDataPoints=1000000  SampleInput=on
  CORDIC_FOFB : Scope  NumInputPorts=2
      settings: TimeRange=0.00011214  YMin=0.475054~-10  YMax=0.52506~45  SaveName=ScopeData5  MaxDataPoints=1000000  SampleInput=on
  bpf_ch0_o{5..8} (4 alike) : xbsIndex_r4/Gateway Out  inherit_from_input=on  hdl_port=off  timing_constraint=Data Rate  locs_specified=off  LOCs={}  UseAsDAC=off  DACChannel='1'  block_type=gatewayout
      settings: infoedit="Gateway out block.  Converts Xilinx fixed-point or floating-point type inputs into ouputs of type Simulink integer, single, double, or fixed point.<br><br>Hardware notes:  In hardware these blocks become top level output ports or are discarded, depending on how they are configured."
  wires:
  bpf_ch0_o5/1 -> CIC_FOFB/1
  [CIC_FOFB_I_FPGA_OUT] -> bpf_ch0_o5/1
  bpf_ch0_o6/1 -> CIC_FOFB/2
  [CIC_FOFB_Q_FPGA_OUT] -> bpf_ch0_o6/1
  bpf_ch0_o7/1 -> CORDIC_FOFB/1
  [CORDIC_FOFB_R_FPGA_OUT] -> bpf_ch0_o7/1
  bpf_ch0_o8/1 -> CORDIC_FOFB/2
  [CORDIC_FOFB_T_FPGA_OUT] -> bpf_ch0_o8/1

== system ddc_bpm_476_066/Channel2_fofb/cic_fofb ==
  Q_in : Inport
  I_in : Inport  Port=2
  Reinterpret : xbsIndex_r4/Reinterpret  force_arith_type=on  arith_type="Signed  (2's comp)"  force_bin_pt=on  bin_pt=22  block_type=reinterpret
  Reinterpret1 : xbsIndex_r4/Reinterpret  force_arith_type=on  arith_type="Signed  (2's comp)"  force_bin_pt=on  bin_pt=22  block_type=reinterpret
  Terminator : Terminator
  Terminator1 : Terminator
  cic_fofb_i : xbsIndex_r4/CIC Compiler 3.0   filter_type=Decimation  number_of_stages=5  differential_delay=2  number_of_channels=1  sample_rate_changes=Fixed  fixed_or_initial_rate=R_fofb  minimum_rate=1113  maximum_rate=1113  ratespecification=Maximum_Possible  sampleperiod=1  hardwareoversamplingrate=1  quantization=Truncation  output_data_width=24  use_xtreme_dsp_slice=on  use_streaming_interface=on  has_aclken=off  has_aresetn=off  has_dout_tready=off  trim_axipin_name=on  gui_behaviour=Sysgen_GUI  input_data_width=18  ip_name=CIC Compiler  ip_version=3.0  dsptool_ready=true  wrapper_available=true  port_translation_map={ 'aclken' => 'en', 'aresetn' => 'rst' }  ipcore_xco_need_fpga_part=true  ipcore_fpga_part=xlipgetpartsetting(gcb, {'virtex7', 'xc7v1500t', '-2', 'fhg1157'})  ipcore_verbose=false  block_type=cic_compiler_v3_0
  cic_fofb_q : xbsIndex_r4/CIC Compiler 3.0   filter_type=Decimation  number_of_stages=5  differential_delay=2  number_of_channels=1  sample_rate_changes=Fixed  fixed_or_initial_rate=R_fofb  minimum_rate=1113  maximum_rate=1113  ratespecification=Maximum_Possible  sampleperiod=1  hardwareoversamplingrate=1  quantization=Truncation  output_data_width=24  use_xtreme_dsp_slice=on  use_streaming_interface=on  has_aclken=off  has_aresetn=off  has_dout_tready=off  trim_axipin_name=on  gui_behaviour=Sysgen_GUI  input_data_width=18  ip_name=CIC Compiler  ip_version=3.0  dsptool_ready=true  wrapper_available=true  port_translation_map={ 'aclken' => 'en', 'aresetn' => 'rst' }  ipcore_xco_need_fpga_part=true  ipcore_fpga_part=xlipgetpartsetting(gcb, {'virtex7', 'xc7v1500t', '-2', 'fhg1157'})  ipcore_verbose=false  block_type=cic_compiler_v3_0
  Q_out : Outport
  Q_valid : Outport  Port=2
  I_out : Outport  Port=3
  I_valid : Outport  Port=4
  wires:
  I_in/1 -> cic_fofb_i/1
  cic_fofb_i/2 -> I_valid/1
  Q_in/1 -> cic_fofb_q/1
  cic_fofb_q/2 -> Q_valid/1
  cic_fofb_i/1 -> Terminator/1
  cic_fofb_q/1 -> Terminator1/1
  Reinterpret/1 -> Q_out/1
  cic_fofb_q/3 -> Reinterpret/1
  Reinterpret1/1 -> I_out/1
  cic_fofb_i/3 -> Reinterpret1/1

== system ddc_bpm_476_066/Channel2_tbt/Analysis ==
  ADC_in1 : Scope
      settings: TimeRange=0.00011214  YMin=-0.1  YMax=0.1  MaxDataPoints=1000000  SampleInput=on
  CORDIC : Scope  NumInputPorts=2
      settings: TimeRange=0.00011214  YMin=0.475054~-10  YMax=0.52506~45  SaveName=ScopeData5  MaxDataPoints=1000000  SampleInput=on
  DECIM_35 : Scope  NumInputPorts=2
      settings: TimeRange=0.00011214  YMin=0.440352~-0.0607492  YMax=0.440353~-0.060745  SaveName=ScopeData4  MaxDataPoints=1000000  SampleInput=on
  MIX : Scope  NumInputPorts=4
      settings: TimeRange=0.00011214  YMin=-0.1~-1.5~-0.002~-1.5  YMax=1~1.5~0.00075~1.5  SaveName=ScopeData2  MaxDataPoints=1000000  SampleInput=on
  bpf_ch0_o{1,3..10} (9 alike) : xbsIndex_r4/Gateway Out  inherit_from_input=on  hdl_port=off  timing_constraint=Data Rate  locs_specified=off  LOCs={}  UseAsDAC=off  DACChannel='1'  block_type=gatewayout
      settings: infoedit="Gateway out block.  Converts Xilinx fixed-point or floating-point type inputs into ouputs of type Simulink integer, single, double, or fixed point.<br><br>Hardware notes:  In hardware these blocks become top level output ports or are discarded, depending on how they are configured."
  wires:
  [BPF_IN] -> bpf_ch0_o1/1
  bpf_ch0_o3/1 -> MIX/1
  [MIX_I_FPGA_OUT] -> bpf_ch0_o3/1
  [MIX_Q_FPGA_OUT] -> bpf_ch0_o4/1
  bpf_ch0_o4/1 -> MIX/3
  [DDS_MSIN_FPGA_OUT] -> bpf_ch0_o9/1
  bpf_ch0_o9/1 -> MIX/2
  [DDS_COS_FPGA_OUT] -> bpf_ch0_o10/1
  bpf_ch0_o10/1 -> MIX/4
  bpf_ch0_o5/1 -> DECIM_35/1
  [DECIM_35_I_FPGA_OUT] -> bpf_ch0_o5/1
  bpf_ch0_o6/1 -> DECIM_35/2
  [DECIM_35_Q_FPGA_OUT] -> bpf_ch0_o6/1
  bpf_ch0_o7/1 -> CORDIC/1
  [CORDIC_R_FPGA_OUT] -> bpf_ch0_o7/1
  bpf_ch0_o8/1 -> CORDIC/2
  [CORDIC_T_FPGA_OUT] -> bpf_ch0_o8/1
  bpf_ch0_o1/1 -> ADC_in1/1

== system ddc_bpm_476_066/Channel2_tbt/DDC ==
  data_in : Inport
  DDS_msine_in : Inport  Port=2
  DDS_cosine_in : Inport  Port=3
  DDS_valid_in : Inport  Port=4
  Constant1 : xbsIndex_r4/Constant  const=1  gui_display_data_type=Boolean  arith_type=Boolean  n_bits=24  bin_pt=22  preci_type=Single  exp_width=8  frac_width=24  explicit_period=on  period=dt_sim  equ=P=C  opselect=C  inp2=PCIN>>17  opr=+  inp1=P  carry=CIN  dbl_ovrd=off  block_type=constant
  Constant2 : xbsIndex_r4/Constant  const=0  gui_display_data_type=Fixed-point  arith_type=Signed (2's comp)  n_bits=24  bin_pt=22  preci_type=Single  exp_width=8  frac_width=24  explicit_period=on  period=dt_sim  equ=P=C  opselect=C  inp2=PCIN>>17  opr=+  inp1=P  carry=CIN  dbl_ovrd=off  block_type=constant
  Mixer : Subsystem
  mix_q_out : Outport
  mix_i_out : Outport  Port=2
  valid_out : Outport  Port=3
  wires:
  Constant1/1 -> Mixer/3(en)
  Constant2/1 -> Mixer/1(din_q)
  DDS_valid_in/1 -> Mixer/4(dds_valid)
  DDS_cosine_in/1 -> Mixer/5(dds_cosine)
  DDS_msine_in/1 -> Mixer/6(dds_msine)
  data_in/1 -> Mixer/2(din_i)
  Mixer/1(Q) -> mix_q_out/1
  Mixer/2(I) -> mix_i_out/1
  Mixer/3(valid_out) -> valid_out/1

== system ddc_bpm_476_066/Channel2_tbt/decim35 ==
  Q_in : Inport
  I_in : Inport  Port=2
  Cast1 : Subsystem
  Cast4 : Subsystem
  "FIR Compiler 6.2 " : xbsIndex_r4/FIR Compiler 6.2   coefficientvector=Hpoly_35.Numerator  coefficient_sets=1  filter_type=Decimation  rate_change_type=Integer  interpolation_rate=1  decimation_rate=decim_factor_poly_35  number_channels=1  ratespecification=Maximum_Possible  sampleperiod=1  hardwareoversamplingrate=4  filter_architecture=Systolic_Multiply_Accumulate  coefficient_reload=off  coefficient_sign=Signed  quantization=Quantize_Only  coefficient_width=16  bestprecision=on  coefficient_fractional_bits=20  coefficient_structure=Inferred  number_paths=2  output_rounding_mode=Convergent_Rounding_to_Even  output_width=24  optimization_goal=Area  data_has_tlast=Not_Required  m_data_has_tready=off  s_data_has_fifo=off  s_data_has_tuser=Not_Required  m_data_has_tuser=Not_Required  s_config_sync_mode=On_Vector  s_config_method=Single  num_reload_slots=1  has_aclken=off  has_aresetn=off  multi_column_support=Disabled  columnconfig='14'  inter_column_pipe_length=4  data_buffer_type=Automatic  coefficient_buffer_type=Automatic  input_buffer_type=Automatic  output_buffer_type=Automatic  preference_for_other_storage=Automatic  trim_axipin_name=on  passband_min=0.0  passband_max=0.5  stopband_min=0.5  stopband_max=1.0  filter_selection=1  gui_behaviour=Sysgen_GUI  data_sign=Signed  data_width=16  data_fractional_bits=0  wrapper_available=true  ip_wrap_arbitrary_binary_point=true  ip_name=FIR Compiler  ip_version=6.2  dsptool_ready=true  ipcore_usecache=true  ipcore_useipmodelcache=true  ipcore_xco_need_fpga_part=true  port_translation_map={ 'aclken' => 'en', 'aresetn' => 'rst' }  run_core_at_system_period=true  ipcore_fpga_part=xlipgetpartsetting(gcb, {'virtex6', 'xc6vlx75t', '-3', 'ff784'})  structural_sim=false  block_type=fir_compiler_v6_2
      settings: infoedit=Maximum Possible : Maximizes oversampling rate. Abstracted input handshake (no s_data_tvalid) and automatic rate propagation.<br>Hardware Oversampling Rate : Specifies oversampling rate relative to the input sample period. Abstracted input handshake (no s_data_tvalid) and automatic rate propagation.<br>Sample Period : Specifies absolute oversampling rate. No input handshake abstraction (exposes s_data_tvalid) and no rate propagation.
  Terminator : Terminator
  Terminator1 : Terminator
  Q_out : Outport
  I_out : Outport  Port=2
  valid_out : Outport  Port=3
  wires:
  Q_in/1 -> "FIR Compiler 6.2 "/1
  "FIR Compiler 6.2 "/2 -> Cast4/2(en), Cast1/2(en)
  "FIR Compiler 6.2 "/3 -> Cast4/1(data_in)
  Cast4/1(out) -> Q_out/1
  "FIR Compiler 6.2 "/4 -> Cast1/1(data_in)
  Cast1/1(out) -> I_out/1
  I_in/1 -> "FIR Compiler 6.2 "/2
  "FIR Compiler 6.2 "/1 -> Terminator/1
  Cast4/2(valid) -> valid_out/1
  Cast1/2(valid) -> Terminator1/1

== system ddc_bpm_476_066/Channel3_fofb/Analysis ==
  CIC_FOFB : Scope  NumInputPorts=2
      settings: TimeRange=0.00011214  YMin=0.440352~-0.0607492  YMax=0.440353~-0.060745  SaveName=ScopeData4  MaxDataPoints=1000000  SampleInput=on
  CORDIC_FOFB : Scope  NumInputPorts=2
      settings: TimeRange=0.00011214  YMin=0.475054~-10  YMax=0.52506~45  SaveName=ScopeData5  MaxDataPoints=1000000  SampleInput=on
  bpf_ch0_o{5..8} (4 alike) : xbsIndex_r4/Gateway Out  inherit_from_input=on  hdl_port=off  timing_constraint=Data Rate  locs_specified=off  LOCs={}  UseAsDAC=off  DACChannel='1'  block_type=gatewayout
      settings: infoedit="Gateway out block.  Converts Xilinx fixed-point or floating-point type inputs into ouputs of type Simulink integer, single, double, or fixed point.<br><br>Hardware notes:  In hardware these blocks become top level output ports or are discarded, depending on how they are configured."
  wires:
  bpf_ch0_o5/1 -> CIC_FOFB/1
  [CIC_FOFB_I_FPGA_OUT] -> bpf_ch0_o5/1
  bpf_ch0_o6/1 -> CIC_FOFB/2
  [CIC_FOFB_Q_FPGA_OUT] -> bpf_ch0_o6/1
  bpf_ch0_o7/1 -> CORDIC_FOFB/1
  [CORDIC_FOFB_R_FPGA_OUT] -> bpf_ch0_o7/1
  bpf_ch0_o8/1 -> CORDIC_FOFB/2
  [CORDIC_FOFB_T_FPGA_OUT] -> bpf_ch0_o8/1

== system ddc_bpm_476_066/Channel3_fofb/cic_fofb ==
  Q_in : Inport
  I_in : Inport  Port=2
  Reinterpret : xbsIndex_r4/Reinterpret  force_arith_type=on  arith_type="Signed  (2's comp)"  force_bin_pt=on  bin_pt=22  block_type=reinterpret
  Reinterpret1 : xbsIndex_r4/Reinterpret  force_arith_type=on  arith_type="Signed  (2's comp)"  force_bin_pt=on  bin_pt=22  block_type=reinterpret
  Terminator : Terminator
  Terminator1 : Terminator
  cic_fofb_i : xbsIndex_r4/CIC Compiler 3.0   filter_type=Decimation  number_of_stages=5  differential_delay=2  number_of_channels=1  sample_rate_changes=Fixed  fixed_or_initial_rate=R_fofb  minimum_rate=1113  maximum_rate=1113  ratespecification=Maximum_Possible  sampleperiod=1  hardwareoversamplingrate=1  quantization=Truncation  output_data_width=24  use_xtreme_dsp_slice=on  use_streaming_interface=on  has_aclken=off  has_aresetn=off  has_dout_tready=off  trim_axipin_name=on  gui_behaviour=Sysgen_GUI  input_data_width=18  ip_name=CIC Compiler  ip_version=3.0  dsptool_ready=true  wrapper_available=true  port_translation_map={ 'aclken' => 'en', 'aresetn' => 'rst' }  ipcore_xco_need_fpga_part=true  ipcore_fpga_part=xlipgetpartsetting(gcb, {'virtex7', 'xc7v1500t', '-2', 'fhg1157'})  ipcore_verbose=false  block_type=cic_compiler_v3_0
  cic_fofb_q : xbsIndex_r4/CIC Compiler 3.0   filter_type=Decimation  number_of_stages=5  differential_delay=2  number_of_channels=1  sample_rate_changes=Fixed  fixed_or_initial_rate=R_fofb  minimum_rate=1113  maximum_rate=1113  ratespecification=Maximum_Possible  sampleperiod=1  hardwareoversamplingrate=1  quantization=Truncation  output_data_width=24  use_xtreme_dsp_slice=on  use_streaming_interface=on  has_aclken=off  has_aresetn=off  has_dout_tready=off  trim_axipin_name=on  gui_behaviour=Sysgen_GUI  input_data_width=18  ip_name=CIC Compiler  ip_version=3.0  dsptool_ready=true  wrapper_available=true  port_translation_map={ 'aclken' => 'en', 'aresetn' => 'rst' }  ipcore_xco_need_fpga_part=true  ipcore_fpga_part=xlipgetpartsetting(gcb, {'virtex7', 'xc7v1500t', '-2', 'fhg1157'})  ipcore_verbose=false  block_type=cic_compiler_v3_0
  Q_out : Outport
  Q_valid : Outport  Port=2
  I_out : Outport  Port=3
  I_valid : Outport  Port=4
  wires:
  I_in/1 -> cic_fofb_i/1
  cic_fofb_i/2 -> I_valid/1
  Q_in/1 -> cic_fofb_q/1
  cic_fofb_q/2 -> Q_valid/1
  cic_fofb_i/1 -> Terminator/1
  cic_fofb_q/1 -> Terminator1/1
  Reinterpret/1 -> Q_out/1
  cic_fofb_q/3 -> Reinterpret/1
  Reinterpret1/1 -> I_out/1
  cic_fofb_i/3 -> Reinterpret1/1
